simulink model "open_loop_CH_model_3_3"  (R2023b)
settings: Solver=ode1  StartTime=0.0  StopTime=10.0  FixedStep=0.001  RelTol=1e-3
settings Model: Creator=sarth  LastModifiedBy=sarth

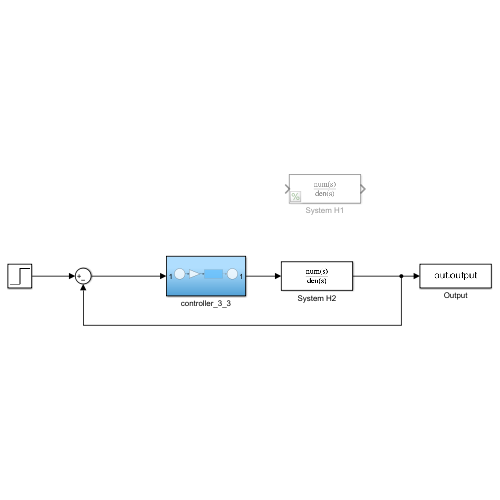
[thumbnail: Simulink's stored preview of the top-level diagram]
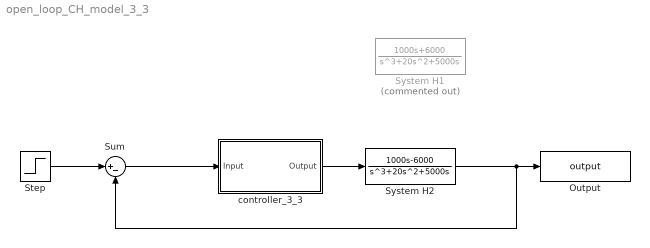
== system open_loop_CH_model_3_3 ==
  Output : ToWorkspace  VariableName=output  SampleTime=-1
  Step : Step  SampleTime=0
  Sum : Sum  Inputs=|+-
  System H1 : TransferFcn  Commented=on  Numerator=[1000 6000]  Denominator=[1 20 5000 0]
  System H2 : TransferFcn  Numerator=[1000 -6000]  Denominator=[1 20 5000 0]
  controller_3_3 : Subsystem
  wires:
  controller_3_3/1(Output) -> System H2/1
  Sum/1 -> controller_3_3/1(Input)
  Step/1 -> Sum/1
  System H2/1 -> Sum/2, Output/1

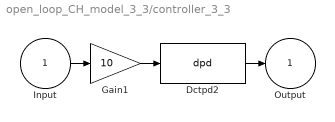
== system open_loop_CH_model_3_3/controller_3_3 ==
  Input : Inport
  Dctpd2 : S-Function  FunctionName=dpd  Parameters=kp, kv, 0.001  SFunctionDeploymentMode=off  EnableBusSupport=off  mask(dctools){kp=2.5, kv=0.01}
      mask help: This block implements a discrete time pd filter.
      mask Display: disp('DCT pd')
  Gain1 : Gain  Gain=10
  Output : Outport
  wires:
  Input/1 -> Gain1/1
  Gain1/1 -> Dctpd2/1
  Dctpd2/1 -> Output/1
